simulink library "import_orbit"  (R2018a)
settings: Solver=VariableStepAuto  StartTime=0.0  StopTime=10.0  RelTol=1e-3
settings Model: Creator=Cédric  LastModifiedBy=Cédric

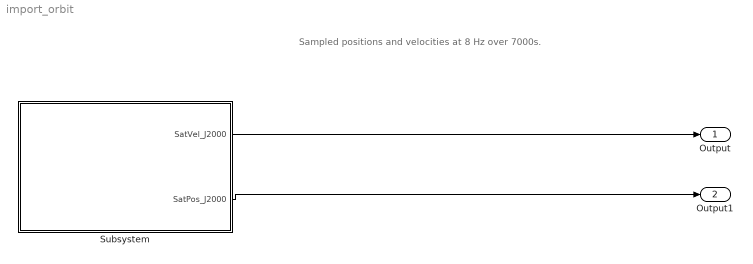
== system import_orbit ==
  note: Sampled positions and velocities at 8 Hz over 7000s.
  Subsystem : Subsystem
  Output : Outport  SignalName=SatVel_J2000
  Output1 : Outport  Port=2  SignalName=SatPos_J2000
  wires:
  Subsystem/2(SatPos_J2000) -> Output1/1
  Subsystem/1(SatVel_J2000) -> Output/1

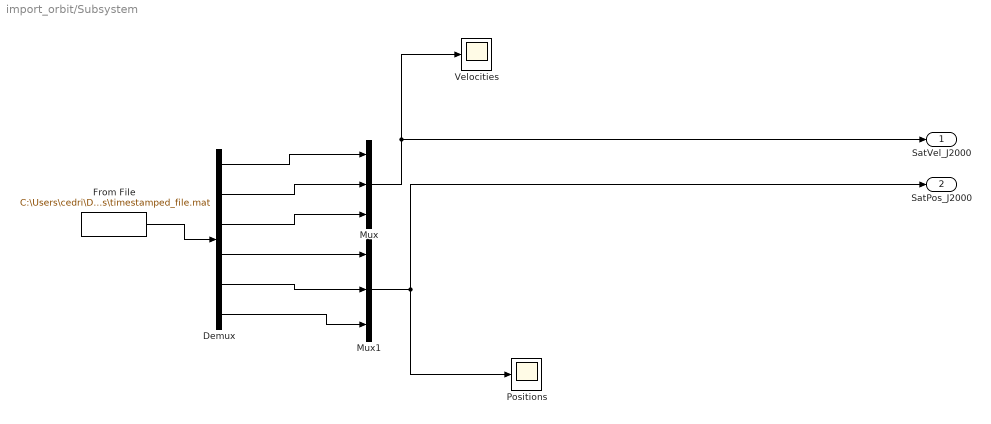
== system import_orbit/Subsystem ==
  Demux : Demux  Outputs=6
  From File : FromFile  FileName=C:\Users\cedri\Documents\TOLOSAT\tolosat_adcs\pythondev\positions\timestamped_file.mat  ExtrapolationBeforeFirstDataPoint=Hold first value  InterpolationWithinTimeRange=Zero order hold  ExtrapolationAfterLastDataPoint=Hold last value
  Mux : Mux  Inputs=3
  Mux1 : Mux  Inputs=3
  Positions : Scope
  Velocities : Scope
  SatVel_J2000 : Outport
  SatPos_J2000 : Outport  Port=2
  wires:
  Demux/5 -> Mux1/2
  Demux/3 -> Mux/3
  Demux/2 -> Mux/2
  Demux/1 -> Mux/1
  Mux/1 -> SatVel_J2000/1, Velocities/1
  From File/1 -> Demux/1
  Demux/4 -> Mux1/1
  Mux1/1 -> SatPos_J2000/1, Positions/1
  Demux/6 -> Mux1/3
